simulink model "gm_pmsm_fpga_slrt"  (R2020b)
settings: Solver=FixedStepDiscrete  StartTime=0.0  StopTime=5  FixedStep=1e-6  RelTol=1e-3
PostLoadFcn:
  | try
  | cell = struct2cell(dir(fullfile(speedgoatroot_hdlb, 'hdlsrc', 'pwm', '*.vhd')));
  | addSourceFiles = strjoin(fullfile(cell(2,:),cell(1,:)), ';');
  | hdlset_param('pwm_example_hdlc/DUT PWM and CAP', 'IPCoreAdditionalFiles', addSourceFiles);
  | end
undefined symbols (not defined in the file or in its folder): FGPA, IO334, pmsm_fpga, Tsc
libraries: speedgoatlib_hdlCoder_IO3xx x12, fl_lib x9, nesl_utility x8, ee_lib x3, slrealtimeutilitieslib x2, pwm_cpulib x1, quadrature_cpulib x1, mcbplantlib x1
settings Model: ModifiedByFormat=Speedgoat GmbH  Creator=Speedgoat GmbH  LastModifiedBy=Speedgoat GmbH
settings SolverCC: ConcurrentTasks=on  PositivePriorityOrder=on
settings DataIOCC: LimitDataPoints=on  SaveFormat=Array  ReturnWorkspaceOutputs=off
settings OptimizationCC: BlockReduction=off  ConditionallyExecuteInputs=off  DefaultParameterBehavior=Inlined  OptimizeBlockIOStorage=off
settings DebuggingCC: AlgebraicLoopMsg=error  UnderspecifiedInitializationDetection=Classic  MergeDetectMultiDrivingBlocksExec=none  SolverPrmCheckMsg=warning  SingleTaskRateTransMsg=error  TasksWithSamePriorityMsg=none  PregeneratedLibrarySubsystemCodeDiagnostic=none  SFUnexpectedBacktrackingDiag=warning  SFNoUnconditionalDefaultTransitionDiag=warning  SFExecutionAtInitializationDiag=none  ArithmeticOperatorsInVariantConditions=warning
settings HardwareCC: ProdBitPerLong=64  ProdLongLongMode=on  ProdHWDeviceType=Intel->x86-64 (Linux 64)
settings ModelReferenceCC: PropagateSignalLabelsOutOfModel=off
settings SFSimCC: SimUseLocalCustomCode=off  CustomCodeUndefinedFunction=UseInterfaceOnly
settings RTWCC: Description=Simulink Real-Time  SystemTargetFile=slrealtime.tlc  TemplateMakefile=slrealtime_default_tmf  RTWUseLocalCustomCode=off  Toolchain=Simulink Real-Time Toolchain  BuildConfiguration=Faster Runs  CodeExecutionProfiling=on  TargetLang=C++
settings CodeAppCC: StateflowObjectComments=on
settings ConfigComp: CovMetricSettings=dw  CovSaveCumulativeToWorkspaceVar=on  CovSaveSingleToWorkspaceVar=on  CovExternalEMLEnable=off

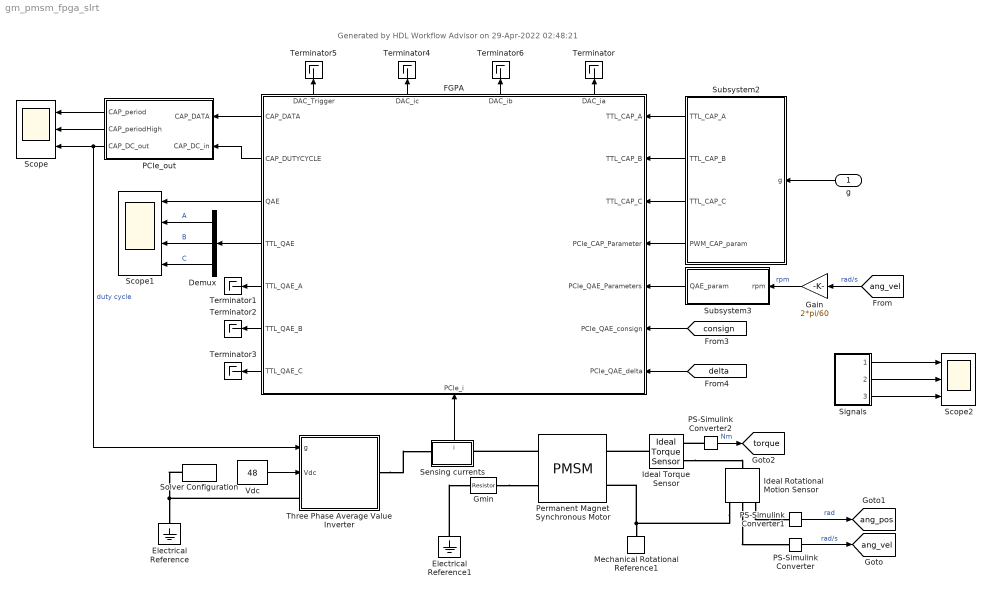
== system gm_pmsm_fpga_slrt ==
  note: Generated by HDL Workflow Advisor on 29-Apr-2022 02:48:21
  g : Inport
  "\t\t\t\t\tFGPA" : Subsystem  mask(Speedgoat IO334-325k Interface Block){module_id=1, slot=-1, ts=-1, OutputRange=Auto (same as ADC), PullRPort0=pull-up 3.3V, VioPort0=3.3V, PullRPort1=pull-up 3.3V, VioPort1=3.3V, PullRPort2=pull-up 3.3V, VioPort2=3.3V, PullRPort3=pull-up 3.3V, VioPort3=3.3V, PullRPort4=pull-up 3.3V, VioPort4=3.3V, PullRPort5=pull-up 3.3V, VioPort5=3.3V, PullRPort6=pull-up 3.3V, VioPort6=3.3V, FpgaFreq=100}
      mask prompts: module_id "FPGA Module Identifier:"; slot "PCI slot (-1: autosearch):"; ts "Sample time:"; OutputRange "DAC Voltage Range:"; PullRPort0 "pull resistor"; VioPort0 "I/O voltage"; PullRPort1 "pull resistor"; VioPort1 "I/O voltage"; PullRPort2 "pull resistor"; VioPort2 "I/O voltage"; PullRPort3 "pull resistor"; VioPort3 "I/O voltage"; PullRPort4 "pull resistor"; VioPort4 "I/O voltage"; PullRPort5 "pull resistor"; VioPort5 "I/O voltage"; PullRPort6 "pull resistor"; VioPort6 "I/O voltage"; FpgaFreq "FPGA Frequency [MHz]"
      mask help: Simulink Real-Time Interface Block for Speedgoat IO334-325k.
      mask init:
      | hdlslrt.backend.mfpgaparameters;
      settings: PortSchema="{\"entries\":[{\"content\":{\"sides\":[{\"content\":{\"connectorIds\":[\"In1\",\"In2\",\"In3\",\"In4\",\"In5\",\"In6\",\"In7\"]},\"type\":\"ConnectorPlacement.EquallySpacedRectSide\",\"uuid\":\"09f41ee4-059e-4ab1-afc0-d52b031ab0c4\"},{\"content\":{\"connectorIds\":[\"Out1\",\"Out2\",\"Out3\",\"Out4\",\"Out5\",\"Out6\",\"Out7\"],\"side\":\"RIGHT\"},\"type\":\"ConnectorPlacement.EquallySpacedRectSide\",\"uuid\":\"926d8c6f-1b97-42bd-ba0a-b1c9c5161ab4\"},{\"content\":{\"connectorIds\":[\"Out8\",\"Out9\",\"Out10\",\"Out11\"],\"side\":\"TOP\"},\"type\":\"ConnectorPlacement.EquallySpacedRectSide\",\"uuid\":\"6ab2c3fb-e2c1-4ae8-b34b-694e17917350\"},{\"content\":{\"connectorIds\":[\"In8\"],\"side\":\"BOTTOM\"},\"type\":\"ConnectorPlacement.EquallySpacedRectSide\",\"uuid\":\"2d5e78c8-9be1-4c52-9ff7-bd20c64ea6bd\"},{\"content\":{\"connectorIds\":[],\"side\":\"HIDDEN\"},\"type\":\"ConnectorPlacement.EquallySpacedRectSide\",\"uuid\":\"a9415aa6-c00d-42bb-a564-ccbbb4bc9464\"}]},\"type\":\"ConnectorPlacement.EquallySpacedConnector\",\"uuid\":\"3d6ab48f-3798-49ac-ac30-1f79e5b6f4e2\"}],\"packageUris\":[\"http://schema.mathworks.com/mf0/Connector/R2020b\"],\"version\":\"1.0\"}"
      mask Help: eval('speedgoatdoc_hdlc')
      mask TypeOptions OutputRange: IO334 DAC Setup/OutputRange
      mask TypeOptions PullRPort0: Port Settings -2x/PullRPort0
      mask Callback PullRPort0: sg_fpga_HDLCoder_io3xx_2x_m(2)
      mask TypeOptions VioPort0: Port Settings -2x/VioPort0
      mask Callback VioPort0: sg_fpga_HDLCoder_io3xx_2x_m(2)
      mask TypeOptions PullRPort1: Port Settings -2x/PullRPort1
      mask Callback PullRPort1: sg_fpga_HDLCoder_io3xx_2x_m(2)
      mask TypeOptions VioPort1: Port Settings -2x/VioPort1
      mask Callback VioPort1: sg_fpga_HDLCoder_io3xx_2x_m(2)
      mask TypeOptions PullRPort2: Port Settings -2x/PullRPort2
      mask Callback PullRPort2: sg_fpga_HDLCoder_io3xx_2x_m(2)
      mask TypeOptions VioPort2: Port Settings -2x/VioPort2
      mask Callback VioPort2: sg_fpga_HDLCoder_io3xx_2x_m(2)
      mask TypeOptions PullRPort3: Port Settings -2x/PullRPort3
      mask Callback PullRPort3: sg_fpga_HDLCoder_io3xx_2x_m(2)
      mask TypeOptions VioPort3: Port Settings -2x/VioPort3
      mask Callback VioPort3: sg_fpga_HDLCoder_io3xx_2x_m(2)
      mask TypeOptions PullRPort4: Port Settings -2x/PullRPort4
      mask Callback PullRPort4: sg_fpga_HDLCoder_io3xx_2x_m(2)
      mask TypeOptions VioPort4: Port Settings -2x/VioPort4
      mask Callback VioPort4: sg_fpga_HDLCoder_io3xx_2x_m(2)
      mask TypeOptions PullRPort5: Port Settings -2x/PullRPort5
      mask Callback PullRPort5: sg_fpga_HDLCoder_io3xx_2x_m(2)
      mask TypeOptions VioPort5: Port Settings -2x/VioPort5
      mask Callback VioPort5: sg_fpga_HDLCoder_io3xx_2x_m(2)
      mask TypeOptions PullRPort6: Port Settings -2x/PullRPort6
      mask Callback PullRPort6: sg_fpga_HDLCoder_io3xx_2x_m(2)
      mask TypeOptions VioPort6: Port Settings -2x/VioPort6
      mask Callback VioPort6: sg_fpga_HDLCoder_io3xx_2x_m(2)
      mask DialogControl AnalogOutput Prompt: Analog Output
      mask DialogControl IO33421 Prompt: IO334-21
      mask DialogControl port1 Prompt: Port 1
      mask DialogControl port2 Prompt: Port 2
      mask DialogControl port3 Prompt: Port 3
      mask DialogControl port4 Prompt: Port 4
      mask DialogControl port5 Prompt: Port 5
      mask DialogControl port6 Prompt: Port 6
      mask DialogControl port7 Prompt: Port 7
      mask Display:
      | SetupBlkPath = find_system(gcb, 'LookUnderMasks', 'all', 'FollowLinks', 'on', 'regexp', 'on', 'Name', 'IO3(\d|x){2}\s+Setup' );
      | SetupBlkPath = SetupBlkPath{1};
      | TS = get_param(SetupBlkPath,'timestamp_mcs');
      | disp(sprintf('Speedgoat IO334-325k\nFPGA I/O Module\n\nTimestamp\n%s\n\nReference Design\nVersion 2.1\n\nMatlab R2020b\n\nPCIe Link Width: X4\nRear Plugin: -21\nAurora Mode: None\nAurora Byteswap: true\n', TS))
  Demux : Demux  Outputs=3
  Electrical Reference : fl_lib/Electrical/Electrical Elements/Electrical Reference
      settings: SourceProductName=Foundation Library
  Electrical Reference1 : fl_lib/Electrical/Electrical Elements/Electrical Reference
      settings: SourceProductName=Foundation Library
  Gain : Gain  Gain=2*pi/60
  Gmin : fl_lib/Electrical/Electrical Elements/Resistor  R=1e6 Ohm  i_specify=off  i_priority=High  i=0 A  i_nominal_specify=off  i_nominal_unit=A  i_nominal_value=1  v_specify=off  v_priority=High  v=0 V  v_nominal_specify=off  v_nominal_unit=V  v_nominal_value=1
      settings: SourceProductName=Foundation Library
  Ideal Rotational Motion Sensor : fl_lib/Mechanical/Mechanical Sensors/Ideal Rotational Motion Sensor  wrap_angle=simscape.enum.onoff.off  offset=0 deg
      settings: SourceProductName=Foundation Library
  Ideal Torque Sensor : fl_lib/Mechanical/Mechanical Sensors/Ideal Torque Sensor
  Mechanical Rotational Reference1 : fl_lib/Mechanical/Rotational Elements/Mechanical Rotational Reference
      settings: SourceProductName=Foundation Library
  PCIe_out : Subsystem
  PS-Simulink Converter : nesl_utility/PS-Simulink Converter  PhysicalDomain=network_engine_domain  SubClassName=ps_output  LeftPortType=input  RightPortType=output  PseudoPeriodic=off  Frequencies=[]  Unit=inherit  AffineConversion=off
  PS-Simulink Converter1 : nesl_utility/PS-Simulink Converter  PhysicalDomain=network_engine_domain  SubClassName=ps_output  LeftPortType=input  RightPortType=output  PseudoPeriodic=off  Frequencies=[]  Unit=inherit  AffineConversion=off
  PS-Simulink Converter2 : nesl_utility/PS-Simulink Converter  PhysicalDomain=network_engine_domain  SubClassName=ps_output  LeftPortType=input  RightPortType=output  PseudoPeriodic=off  Frequencies=[]  Unit=inherit  AffineConversion=off
  Permanent Magnet Synchronous Motor : ee_lib/Electromechanical/Permanent Magnet/PMSM  winding_type=ee.enum.statorconnection.wye  machine_param=ee.enum.pmsm.parameterization.constant  nPolePairs=N  pmflux_param=ee.enum.pmflux.fluxlinkage  pm_flux_linkage=PM Wb  torque_constant=0.18 N*m/A  back_emf_constant=0.18 V/(rad/s)  stator_param=ee.enum.statorparam.LdLqL0  Ld=Ld H  Lq=Lq H  idVec=[-200, 0, 200] A  iqVec=[-200, 0, 200] A  LdMatrix=0.0002 * ones(3, 3) H  LqMatrix=0.0002 * ones(3, 3) H  PmMatrix=0.1 * ones(3, 3) Wb  ktMatrix=0.18 * ones(3, 3) N*m/A  keMatrix=0.18 * ones(3, 3) V/(rad/s)  L0=L0 H  Ls=0.0002 H  Lm=0.00002 H  Ms=0.00002 H  Rs=Rs Ohm  zero_sequence=ee.enum.park.zerosequence.exclude  J=0 kg*m^2  lam=0 N*m/(rad/s)  axes_param=ee.enum.rotorangle.qaxis  i_d_specify=off  i_d_priority=None  i_d=0 A  i_d_nominal_specify=off  i_d_nominal_unit=A  i_d_nominal_value=1  i_q_specify=off  i_q_priority=None  i_q=0 A  i_q_nominal_specify=off  i_q_nominal_unit=A  i_q_nominal_value=1  torque_specify=off  torque_priority=None  torque=0 N*m  torque_nominal_specify=off  torque_nominal_unit=N*m  torque_nominal_value=1  angular_velocity_specify=on  angular_velocity_priority=None  angular_velocity=0 rpm  angular_velocity_nominal_specify=off  angular_velocity_nominal_unit=rpm  angular_velocity_nominal_value=1  angular_position_specify=on  angular_position_priority=High  angular_position=0 rad  angular_position_nominal_specify=off  angular_position_nominal_unit=deg  angular_position_nominal_value=1  loss_param=ee.enum.ironloss.none  losses_oc=[0, 0, 0] W  losses_sc=[0, 0, 0] W  f_losses=60 Hz  Isc_losses=95 A  Tmeas=298.15 K  alpha=3.93e-3 1/K  alpha_flux=-0.001 1/K  stator_thermal_mass=100 J/K  rotor_thermal_mass=200 J/K  Rm_percent_rotor=90  Rd_percent_rotor=30  temperatureA_specify=off  temperatureA_priority=High  temperatureA=25 degC  temperatureA_nominal_specify=off  temperatureA_nominal_unit=degC  temperatureA_nominal_value=1  temperatureB_specify=off  temperatureB_priority=High  temperatureB=25 degC  temperatureB_nominal_specify=off  temperatureB_nominal_unit=degC  temperatureB_nominal_value=1  temperatureC_specify=off  temperatureC_priority=High  temperatureC=25 degC  temperatureC_nominal_specify=off  temperatureC_nominal_unit=degC  temperatureC_nominal_value=1  temperatureR_specify=off  temperatureR_priority=High  temperatureR=25 degC  temperatureR_nominal_specify=off  temperatureR_nominal_unit=degC  temperatureR_nominal_value=1
      settings: SourceProductName=Electrical  InternalSimscapePortConfiguration="{\"Bottom\":[],\"Left\":[{\"id\":\"N\",\"label\":\"~\",\"type\":\"foundation.electrical.three_phase\"},{\"id\":\"n\",\"label\":\"n\",\"type\":\"foundation.electrical.electrical\"}],\"Right\":[{\"id\":\"R\",\"label\":\"R\",\"type\":\"foundation.mechanical.rotational.rotational\"},{\"id\":\"C\",\"label\":\"C\",\"type\":\"foundation.mechanical.rotational.rotational\"}],\"Top\":[]}"
  Scope : Scope  NumInputPorts=3
  Scope1 : Scope  NumInputPorts=4
  Scope2 : Scope  NumInputPorts=3
  Sensing currents : Subsystem
      settings: PortSchema="{\"entries\":[{\"content\":{\"sides\":[{\"content\":{\"connectorIds\":[\"LConn1\"]},\"type\":\"ConnectorPlacement.EquallySpacedRectSide\",\"uuid\":\"1aa2d636-2edb-4c6c-8a85-076f6d921b68\"},{\"content\":{\"connectorIds\":[\"RConn1\"],\"side\":\"RIGHT\"},\"type\":\"ConnectorPlacement.EquallySpacedRectSide\",\"uuid\":\"a6523212-cffe-411b-b118-58c3b70b54bd\"},{\"content\":{\"connectorIds\":[\"Out1\"],\"side\":\"TOP\"},\"type\":\"ConnectorPlacement.EquallySpacedRectSide\",\"uuid\":\"99131e59-73db-485e-9354-6c0d4554cf91\"},{\"content\":{\"connectorIds\":[],\"side\":\"HIDDEN\"},\"type\":\"ConnectorPlacement.EquallySpacedRectSide\",\"uuid\":\"e90ddb90-c2ae-41a5-978d-aaeb282058ac\"}]},\"type\":\"ConnectorPlacement.EquallySpacedConnector\",\"uuid\":\"53267539-7307-4a2c-98d0-de38e9871156\"}],\"packageUris\":[\"http://schema.mathworks.com/mf0/Connector/R2020b\"],\"version\":\"1.0\"}"
      mask Display: disp('i')
  Signals : Subsystem
  Solver Configuration : nesl_utility/Solver Configuration  PhysicalDomain=network_engine_domain  SubClassName=solver  LeftPortType=input  RightPortType=generic  Tones=[]  Harmonics=[]  SimulateNoise=off  Profile=off  UseLocalSampling=off  EnableSwitchedLinearOptims=on  FrequencyDomain=off  UseCCode=off  RelTol=0.001  AbsTol=1e-06  MinStep=1e-09  ToWorkspace=off  RevertToSquareIcSolve=off  NumHomotopyIterations=100  PhasorMode=off  PhasorModeNumHarmonics=1  DoDC=off  ResidualTolerance=1e-9  UseLocalSolver=on  LocalSolverChoice=NE_BACKWARD_EULER_ADVANCER  LocalSolverSampleTime=Ts  DoFixedCost=on  MaxNonlinIter=4  MaxModeIter=2  ComputeImpulses=off  ImpulseIterations=2  LinearAlgebra=auto  EquationFormulation=NE_TIME_EF  DelaysMemoryBudget=1024  AutomaticFiltering=on  FilteringTimeConstant=0.001  PartitionStorageMethod=AS_NEEDED  PartitionMemoryBudget=1024  PartitionMethod=FAST
      settings: SourceProductName=Utilities
  Subsystem2 : Subsystem
  Subsystem3 : Subsystem
  Terminator{,1..6} (7 alike) : Terminator
  Three Phase Average Value Inverter : Subsystem
  Vdc : Constant  Value=48  SampleTime=Tsc
  tag scope: ang_pos=global, ang_vel=global, torque=global
  wires:
  Demux/3 -> Scope1/4  "C"
  Demux/1 -> Scope1/2  "A"
  Demux/2 -> Scope1/3  "B"
  "\t\t\t\t\tFGPA"/4(TTL_QAE) -> Demux/1
  "\t\t\t\t\tFGPA"/3(QAE) -> Scope1/1
  "\t\t\t\t\tFGPA"/10(DAC_ic) -> Terminator4/1
  "\t\t\t\t\tFGPA"/11(DAC_Trigger) -> Terminator5/1
  "\t\t\t\t\tFGPA"/9(DAC_ib) -> Terminator6/1
  Signals/3(ang_vel) -> Scope2/3
  Signals/2(ang_pos) -> Scope2/2
  Signals/1(torque) -> Scope2/1
  PS-Simulink Converter1/1 -> [ang_pos]  "rad"
  PS-Simulink Converter2/1 -> [torque]  "Nm"
  [ang_vel] -> Gain/1  "rad/s"
  Gain/1 -> Subsystem3/1(rpm)  "rpm"
  PS-Simulink Converter/1 -> [ang_vel]  "rad/s"
  Sensing currents/1(i) -> "\t\t\t\t\tFGPA"/8(PCIe_i)
  "\t\t\t\t\tFGPA"/8(DAC_ia) -> Terminator/1
  "\t\t\t\t\tFGPA"/7(TTL_QAE_C) -> Terminator3/1
  "\t\t\t\t\tFGPA"/6(TTL_QAE_B) -> Terminator2/1
  "\t\t\t\t\tFGPA"/5(TTL_QAE_A) -> Terminator1/1
  "\t\t\t\t\tFGPA"/2(CAP_DUTYCYCLE) -> PCIe_out/2(CAP_DC_in)
  "\t\t\t\t\tFGPA"/1(CAP_DATA) -> PCIe_out/1(CAP_DATA)
  [delta] -> "\t\t\t\t\tFGPA"/7(PCIe_QAE_delta)
  [consign] -> "\t\t\t\t\tFGPA"/6(PCIe_QAE_consign)
  Subsystem3/1(QAE_param) -> "\t\t\t\t\tFGPA"/5(PCIe_QAE_Parameters)
  Subsystem2/4(PWM_CAP_param) -> "\t\t\t\t\tFGPA"/4(PCIe_CAP_Parameter)
  Subsystem2/3(TTL_CAP_C) -> "\t\t\t\t\tFGPA"/3(TTL_CAP_C)
  Subsystem2/2(TTL_CAP_B) -> "\t\t\t\t\tFGPA"/2(TTL_CAP_B)
  Subsystem2/1(TTL_CAP_A) -> "\t\t\t\t\tFGPA"/1(TTL_CAP_A)
  PCIe_out/3(CAP_DC_out) -> Three Phase Average Value Inverter/1(g), Scope/3  "duty cycle"
  g/1 -> Subsystem2/1(g)
  Vdc/1 -> Three Phase Average Value Inverter/2(Vdc)
  PCIe_out/1(CAP_period) -> Scope/1
  PCIe_out/2(CAP_periodHigh) -> Scope/2
  connections:
  PS-Simulink Converter2/LConn1 -- Ideal Torque Sensor/RConn2
  Ideal Torque Sensor/RConn1 -- Ideal Rotational Motion Sensor/LConn1
  Ideal Torque Sensor/LConn1 -- Permanent Magnet Synchronous Motor/RConn1
  Ideal Rotational Motion Sensor/RConn3 -- PS-Simulink Converter1/LConn1
  Ideal Rotational Motion Sensor/RConn2 -- PS-Simulink Converter/LConn1
  Solver Configuration/RConn1 -- Electrical Reference/LConn1 -- Three Phase Average Value Inverter/LConn1
  Electrical Reference1/LConn1 -- Gmin/LConn1
  Permanent Magnet Synchronous Motor/LConn1 -- Sensing currents/RConn1
  Three Phase Average Value Inverter/RConn1 -- Sensing currents/LConn1
  Gmin/RConn1 -- Permanent Magnet Synchronous Motor/LConn2
  Ideal Rotational Motion Sensor/RConn1 -- Permanent Magnet Synchronous Motor/RConn2 -- Mechanical Rotational Reference1/LConn1

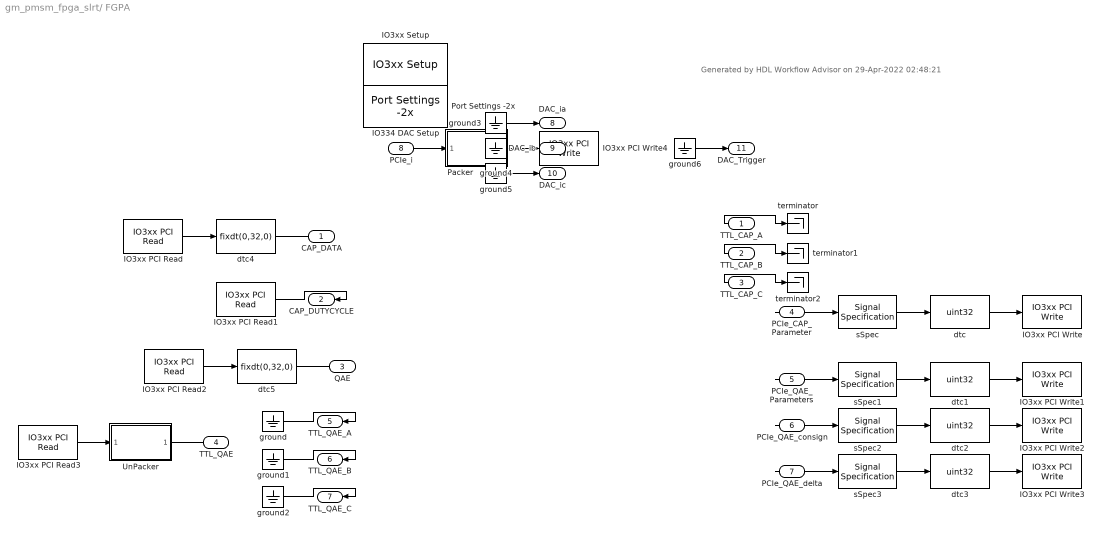
== system gm_pmsm_fpga_slrt/					FGPA ==
  note: Generated by HDL Workflow Advisor on 29-Apr-2022 02:48:21
  TTL_CAP_A : Inport
  TTL_CAP_B : Inport  Port=2
  TTL_CAP_C : Inport  Port=3
  PCIe_CAP_Parameter : Inport  Port=4
  PCIe_QAE_Parameters : Inport  Port=5
  PCIe_QAE_consign : Inport  Port=6
  PCIe_QAE_delta : Inport  Port=7
  PCIe_i : Inport  Port=8
  IO334 DAC Setup : speedgoatlib_hdlCoder_IO3xx/IO334 DAC Setup  module_id=module_id  OutputRange=Auto (same as ADC)
  IO3xx PCI Read : speedgoatlib_hdlCoder_IO3xx/IO3xx PCI Read  device_id=deviceIdx  module_id=module_id  board_type=IO3xx  port_name=CAP_DATA  port_offset=hex2dec('180')  port_type=uint32  port_dim=18  strobe=hex2dec('200')  sample_time=ts
  IO3xx PCI Read1 : speedgoatlib_hdlCoder_IO3xx/IO3xx PCI Read  device_id=deviceIdx  module_id=module_id  board_type=IO3xx  port_name=CAP_DUTYCYCLE  port_offset=hex2dec('160')  port_type=single  port_dim=3  strobe=hex2dec('170')  sample_time=ts
  IO3xx PCI Read2 : speedgoatlib_hdlCoder_IO3xx/IO3xx PCI Read  device_id=deviceIdx  module_id=module_id  board_type=IO3xx  port_name=QAE  port_offset=hex2dec('11C')  port_type=uint32  port_dim=1  strobe=0  sample_time=ts
  IO3xx PCI Read3 : speedgoatlib_hdlCoder_IO3xx/IO3xx PCI Read  device_id=deviceIdx  module_id=module_id  board_type=IO3xx  port_name=TTL_QAE  port_offset=hex2dec('144')  port_type=uint32  port_dim=1  strobe=0  sample_time=ts
  IO3xx PCI Write : speedgoatlib_hdlCoder_IO3xx/IO3xx PCI Write  device_id=deviceIdx  module_id=module_id  board_type=IO3xx  port_name=PCIe_CAP_Parameter  port_offset=hex2dec('100')  port_type=uint32  port_dim=3  strobe=hex2dec('110')  sample_time=ts
  IO3xx PCI Write1 : speedgoatlib_hdlCoder_IO3xx/IO3xx PCI Write  device_id=deviceIdx  module_id=module_id  board_type=IO3xx  port_name=PCIe_QAE_Parameters  port_offset=hex2dec('120')  port_type=uint32  port_dim=7  strobe=hex2dec('140')  sample_time=ts
  IO3xx PCI Write2 : speedgoatlib_hdlCoder_IO3xx/IO3xx PCI Write  device_id=deviceIdx  module_id=module_id  board_type=IO3xx  port_name=PCIe_QAE_consign  port_offset=hex2dec('114')  port_type=uint32  port_dim=1  strobe=0  sample_time=ts
  IO3xx PCI Write3 : speedgoatlib_hdlCoder_IO3xx/IO3xx PCI Write  device_id=deviceIdx  module_id=module_id  board_type=IO3xx  port_name=PCIe_QAE_delta  port_offset=hex2dec('118')  port_type=uint32  port_dim=1  strobe=0  sample_time=ts
  IO3xx PCI Write4 : speedgoatlib_hdlCoder_IO3xx/IO3xx PCI Write  device_id=deviceIdx  module_id=module_id  board_type=IO3xx  port_name=PCIe_i  port_offset=hex2dec('148')  port_type=uint32  port_dim=2  strobe=hex2dec('150')  sample_time=ts
  IO3xx Setup : speedgoatlib_hdlCoder_IO3xx/IO3xx Setup  mdl_ss_name="pmsm_fpga/\t\t\t\t\tFGPA"  board_type=IO334-325k  fpga_sync_mode=on  reset_mode=on  device_id=deviceIdx  module_id=module_id  pci_slot=slot  fpga_mat_file=hdl_prj\hdlsrc\pmsm_fpga\FGPA.mat  timestamp_mcs=04/29/22 02:35:43  timestamp=2204290144  tsreg=hex2dec('8')  bsf_file=FGPA_2204290144.mcs  mcs=0
  Packer : Subsystem
  Port Settings -2x : speedgoatlib_hdlCoder_IO3xx/Port Settings -2x  module_id=module_id  rearIO=-21  PullRPort0=pull-up 3.3V  VioPort0=3.3V  PullRPort1=pull-up 3.3V  VioPort1=3.3V  PullRPort2=pull-up 3.3V  VioPort2=3.3V  PullRPort3=pull-up 3.3V  VioPort3=3.3V  PullRPort4=pull-up 3.3V  VioPort4=3.3V  PullRPort5=pull-up 3.3V  VioPort5=3.3V  PullRPort6=pull-up 3.3V  VioPort6=3.3V
  UnPacker : Subsystem
  dtc{,1..3} (4 alike) : DataTypeConversion  OutDataTypeStr=uint32  ConvertRealWorld=Stored Integer (SI)  RndMeth=Zero
  dtc4 : DataTypeConversion  OutDataTypeStr=fixdt(0,32,0)  ConvertRealWorld=Stored Integer (SI)  RndMeth=Zero
  dtc5 : DataTypeConversion  OutDataTypeStr=fixdt(0,32,0)  ConvertRealWorld=Stored Integer (SI)  RndMeth=Zero
  ground{,1..6} (7 alike) : Ground
  sSpec : SignalSpecification  OutDataTypeStr=fixdt(0,32,0)
  sSpec1 : SignalSpecification  OutDataTypeStr=fixdt(0,32,0)
  sSpec2 : SignalSpecification  OutDataTypeStr=fixdt(0,32,0)
  sSpec3 : SignalSpecification  OutDataTypeStr=fixdt(1,32,0)
  terminator : Terminator
  terminator1 : Terminator
  terminator2 : Terminator
  CAP_DATA : Outport
  CAP_DUTYCYCLE : Outport  Port=2
  QAE : Outport  Port=3
  TTL_QAE : Outport  Port=4
  TTL_QAE_A : Outport  Port=5
  TTL_QAE_B : Outport  Port=6
  TTL_QAE_C : Outport  Port=7
  DAC_ia : Outport  Port=8
  DAC_ib : Outport  Port=9
  DAC_ic : Outport  Port=10
  DAC_Trigger : Outport  Port=11
  wires:
  TTL_CAP_A/1 -> terminator/1
  TTL_CAP_B/1 -> terminator1/1
  TTL_CAP_C/1 -> terminator2/1
  PCIe_CAP_Parameter/1 -> sSpec/1
  sSpec/1 -> dtc/1
  dtc/1 -> IO3xx PCI Write/1
  PCIe_QAE_Parameters/1 -> sSpec1/1
  sSpec1/1 -> dtc1/1
  dtc1/1 -> IO3xx PCI Write1/1
  PCIe_QAE_consign/1 -> sSpec2/1
  sSpec2/1 -> dtc2/1
  dtc2/1 -> IO3xx PCI Write2/1
  PCIe_QAE_delta/1 -> sSpec3/1
  sSpec3/1 -> dtc3/1
  dtc3/1 -> IO3xx PCI Write3/1
  PCIe_i/1 -> Packer/1(unpacked)
  Packer/1(packed) -> IO3xx PCI Write4/1
  dtc4/1 -> CAP_DATA/1
  IO3xx PCI Read/1 -> dtc4/1
  IO3xx PCI Read1/1 -> CAP_DUTYCYCLE/1
  dtc5/1 -> QAE/1
  IO3xx PCI Read2/1 -> dtc5/1
  UnPacker/1(unpacked) -> TTL_QAE/1
  IO3xx PCI Read3/1 -> UnPacker/1(packed)
  ground/1 -> TTL_QAE_A/1
  ground1/1 -> TTL_QAE_B/1
  ground2/1 -> TTL_QAE_C/1
  ground3/1 -> DAC_ia/1
  ground4/1 -> DAC_ib/1
  ground5/1 -> DAC_ic/1
  ground6/1 -> DAC_Trigger/1

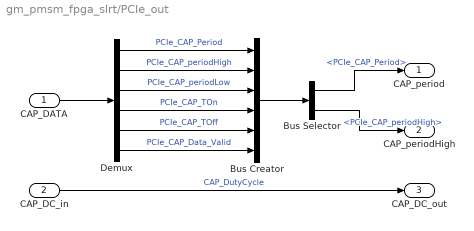
== system gm_pmsm_fpga_slrt/PCIe_out ==
  CAP_DATA : Inport
  CAP_DC_in : Inport  Port=2
  Bus Creator : BusCreator  Inputs=6
  Bus Selector : BusSelector  OutputSignals=PCIe_CAP_Period,PCIe_CAP_periodHigh
  Demux : Demux  Outputs=6
  CAP_period : Outport
  CAP_periodHigh : Outport  Port=2
  CAP_DC_out : Outport  Port=3
  wires:
  CAP_DATA/1 -> Demux/1
  Demux/5 -> Bus Creator/5  "PCIe_CAP_TOff"
  Demux/1 -> Bus Creator/1  "PCIe_CAP_Period"
  Bus Creator/1 -> Bus Selector/1
  Demux/4 -> Bus Creator/4  "PCIe_CAP_TOn"
  Demux/2 -> Bus Creator/2  "PCIe_CAP_periodHigh"
  Demux/3 -> Bus Creator/3  "PCIe_CAP_periodLow"
  Demux/6 -> Bus Creator/6  "PCIe_CAP_Data_Valid"
  Bus Selector/1 -> CAP_period/1  "<PCIe_CAP_Period>"
  Bus Selector/2 -> CAP_periodHigh/1  "<PCIe_CAP_periodHigh>"
  CAP_DC_in/1 -> CAP_DC_out/1  "CAP_DutyCycle"

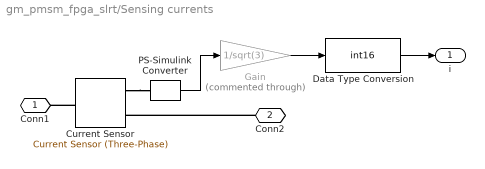
== system gm_pmsm_fpga_slrt/Sensing currents ==
  Current Sensor : ee_lib/Sensors & Transducers/Current Sensor (Three-Phase)
      settings: SourceProductName=Electrical
  Data Type Conversion : DataTypeConversion  OutDataTypeStr=int16
  Gain : Gain  Commented=through  Gain=1/sqrt(3)
  PS-Simulink Converter : nesl_utility/PS-Simulink Converter  PhysicalDomain=network_engine_domain  SubClassName=ps_output  LeftPortType=input  RightPortType=output  PseudoPeriodic=off  Frequencies=[]  Unit=A  AffineConversion=off
      settings: SourceProductName=Utilities
  Conn1 : PMIOPort  Side=Left
  Conn2 : PMIOPort  Port=2  Side=Right
  i : Outport
  wires:
  Gain/1 -> Data Type Conversion/1
  Data Type Conversion/1 -> i/1
  PS-Simulink Converter/1 -> Gain/1
  connections:
  Current Sensor/LConn1 -- Conn1/RConn1
  Conn2/RConn1 -- Current Sensor/RConn2
  Current Sensor/RConn1 -- PS-Simulink Converter/LConn1

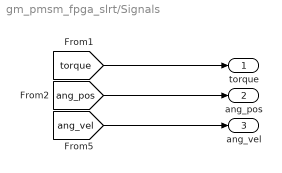
== system gm_pmsm_fpga_slrt/Signals ==
  torque : Outport
  ang_pos : Outport  Port=2
  ang_vel : Outport  Port=3
  wires:
  [ang_pos] -> ang_pos/1
  [ang_vel] -> ang_vel/1
  [torque] -> torque/1

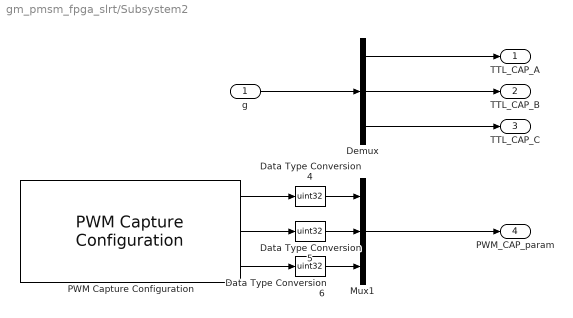
== system gm_pmsm_fpga_slrt/Subsystem2 ==
  g : Inport
  Data Type Conversion4 : DataTypeConversion  OutDataTypeStr=uint32
  Data Type Conversion5 : DataTypeConversion  OutDataTypeStr=uint32
  Data Type Conversion6 : DataTypeConversion  OutDataTypeStr=uint32
  Demux : Demux  Outputs=3
  Mux1 : Mux  Inputs=3
  PWM Capture Configuration : pwm_cpulib/PWM Capture Configuration  FPGA_freq=100e6  n_channels=1  captureMode=High transitions triggered  captureTimeout=0  PWM_pattern_en=off
      settings: SourceProductName=Simulink Real-Time: Speedgoat HDL Blockset
  TTL_CAP_A : Outport
  TTL_CAP_B : Outport  Port=2
  TTL_CAP_C : Outport  Port=3
  PWM_CAP_param : Outport  Port=4
  wires:
  Demux/3 -> TTL_CAP_C/1
  g/1 -> Demux/1
  Data Type Conversion5/1 -> Mux1/2
  Data Type Conversion6/1 -> Mux1/3
  Data Type Conversion4/1 -> Mux1/1
  PWM Capture Configuration/3 -> Data Type Conversion6/1
  PWM Capture Configuration/1 -> Data Type Conversion4/1
  PWM Capture Configuration/2 -> Data Type Conversion5/1
  Demux/2 -> TTL_CAP_B/1
  Mux1/1 -> PWM_CAP_param/1
  Demux/1 -> TTL_CAP_A/1

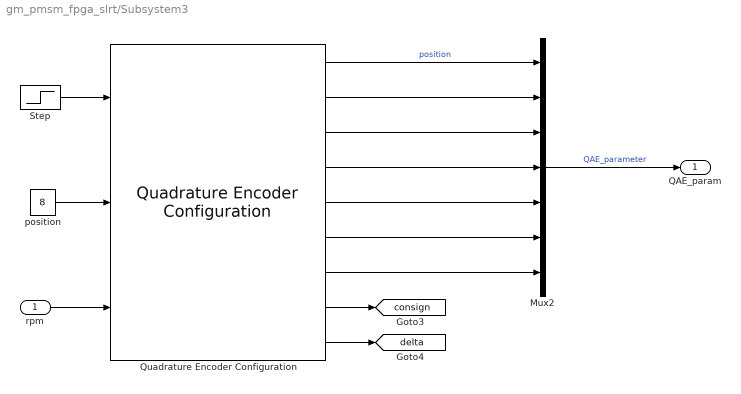
== system gm_pmsm_fpga_slrt/Subsystem3 ==
  rpm : Inport
  Mux2 : Mux  Inputs=7
  Quadrature Encoder Configuration : quadrature_cpulib/Quadrature Encoder Configuration  fpgaFreq=100e6  n_channels=1  numSeg=[16]  phaseAngle=90  initPos=[0]  freeWheel=on
      settings: SourceProductName=Simulink Real-Time: Speedgoat HDL Blockset
  Step : Step  Time=0.002
  position : Constant  Value=8  SampleTime=-1
  QAE_param : Outport
  tag scope: consign=global, delta=global
  wires:
  rpm/1 -> Quadrature Encoder Configuration/3
  position/1 -> Quadrature Encoder Configuration/2
  Quadrature Encoder Configuration/4 -> Mux2/4
  Mux2/1 -> QAE_param/1  "QAE_parameter"
  Quadrature Encoder Configuration/2 -> Mux2/2
  Quadrature Encoder Configuration/8 -> [consign]
  Quadrature Encoder Configuration/9 -> [delta]
  Step/1 -> Quadrature Encoder Configuration/1
  Quadrature Encoder Configuration/7 -> Mux2/7
  Quadrature Encoder Configuration/1 -> Mux2/1  "position"
  Quadrature Encoder Configuration/3 -> Mux2/3
  Quadrature Encoder Configuration/5 -> Mux2/5
  Quadrature Encoder Configuration/6 -> Mux2/6

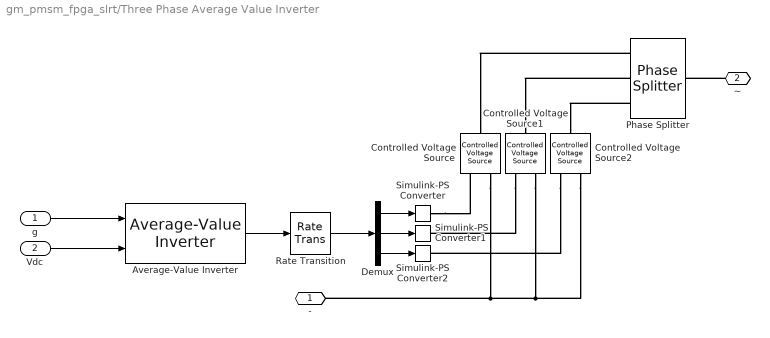
== system gm_pmsm_fpga_slrt/Three Phase Average Value Inverter ==
  g : Inport
  Vdc : Inport  Port=2
  Average-Value Inverter : mcbplantlib/Average-Value Inverter
  Controlled Voltage Source : fl_lib/Electrical/Electrical Sources/Controlled Voltage Source
  Controlled Voltage Source1 : fl_lib/Electrical/Electrical Sources/Controlled Voltage Source
  Controlled Voltage Source2 : fl_lib/Electrical/Electrical Sources/Controlled Voltage Source
  Demux : Demux  Outputs=3
  Phase Splitter : ee_lib/Connectors & References/Phase Splitter
      settings: SourceProductBaseCode=PS
  Rate Transition : RateTransition
  Simulink-PS Converter : nesl_utility/Simulink-PS Converter  PhysicalDomain=network_engine_domain  SubClassName=ps_input  LeftPortType=input  RightPortType=output  PseudoPeriodic=off  Frequencies=[]  NoiseDistribution=none  NoiseParameters=[]  Unit=1  AffineConversion=off  FilteringAndDerivatives=provide  SimscapeFilterOrder=1  InputFilterTimeConstant=0.001  UdotUserProvided=0
  Simulink-PS Converter1 : nesl_utility/Simulink-PS Converter  PhysicalDomain=network_engine_domain  SubClassName=ps_input  LeftPortType=input  RightPortType=output  PseudoPeriodic=off  Frequencies=[]  NoiseDistribution=none  NoiseParameters=[]  Unit=1  AffineConversion=off  FilteringAndDerivatives=provide  SimscapeFilterOrder=1  InputFilterTimeConstant=0.001  UdotUserProvided=0
  Simulink-PS Converter2 : nesl_utility/Simulink-PS Converter  PhysicalDomain=network_engine_domain  SubClassName=ps_input  LeftPortType=input  RightPortType=output  PseudoPeriodic=off  Frequencies=[]  NoiseDistribution=none  NoiseParameters=[]  Unit=1  AffineConversion=off  FilteringAndDerivatives=provide  SimscapeFilterOrder=1  InputFilterTimeConstant=0.001  UdotUserProvided=0
  - : PMIOPort  Tag=PMCPort  Side=Left
  ~ : PMIOPort  Tag=PMCPort  Port=2  Side=Right
  wires:
  Average-Value Inverter/1 -> Rate Transition/1
  Rate Transition/1 -> Demux/1
  g/1 -> Average-Value Inverter/1
  Demux/1 -> Simulink-PS Converter/1
  Demux/2 -> Simulink-PS Converter1/1
  Vdc/1 -> Average-Value Inverter/2
  Demux/3 -> Simulink-PS Converter2/1
  connections:
  Controlled Voltage Source1/RConn1 -- Simulink-PS Converter1/RConn1
  Phase Splitter/RConn2 -- Controlled Voltage Source1/LConn1
  Phase Splitter/RConn1 -- Controlled Voltage Source/LConn1
  Phase Splitter/RConn3 -- Controlled Voltage Source2/LConn1
  Controlled Voltage Source2/RConn1 -- Simulink-PS Converter2/RConn1
  Simulink-PS Converter/RConn1 -- Controlled Voltage Source/RConn1
  Controlled Voltage Source2/RConn2 -- Controlled Voltage Source1/RConn2 -- -/RConn1 -- Controlled Voltage Source/RConn2
  ~/RConn1 -- Phase Splitter/LConn1

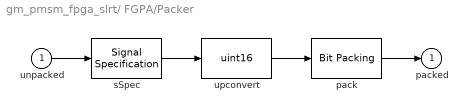
== system gm_pmsm_fpga_slrt/					FGPA/Packer ==
  unpacked : Inport
  pack : slrealtimeutilitieslib/Bit Packing  MaskBitPatterns={[0:15 16:31 32:47 ]}  MaskPackDataType=uint32  MaskPackDataSize=2
      settings: SourceProductBaseCode=XP
  sSpec : SignalSpecification  OutDataTypeStr=fixdt(1,16,0)
  upconvert : DataTypeConversion  OutDataTypeStr=uint16  ConvertRealWorld=Stored Integer (SI)  RndMeth=Zero
  packed : Outport
  wires:
  unpacked/1 -> sSpec/1
  sSpec/1 -> upconvert/1
  upconvert/1 -> pack/1
  pack/1 -> packed/1

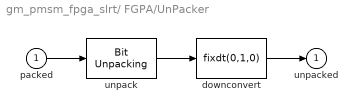
== system gm_pmsm_fpga_slrt/					FGPA/UnPacker ==
  packed : Inport
  downconvert : DataTypeConversion  OutDataTypeStr=fixdt(0,1,0)  ConvertRealWorld=Stored Integer (SI)  RndMeth=Zero
  unpack : slrealtimeutilitieslib/Bit Unpacking  SignExtend=on  MaskBitPatterns={[0:0 -1 -1 -1 -1 -1 -1 -1 1:1 -1 -1 -1 -1 -1 -1 -1 2:2 -1 -1 -1 -1 -1 -1 -1 ]}  MaskPackDataType=uint32  MaskPackDataSize=1  MaskUnpackDataTypes={'uint8'}  MaskUnpackDataSizes={3}
      settings: SourceProductBaseCode=XP
  unpacked : Outport
  wires:
  packed/1 -> unpack/1
  unpack/1 -> downconvert/1
  downconvert/1 -> unpacked/1
